simulink model "vibrationAbsorber"  (R2020b)
settings: Solver=VariableStepAuto  StartTime=0.0  StopTime=50  RelTol=1e-3
PreLoadFcn:
  | M1 = 100;
  | K1 = 50;
  | b = 50;
  | K12 = 500;
  | M2 = 5;
settings Model: Creator=Admin  LastModifiedBy=Admin

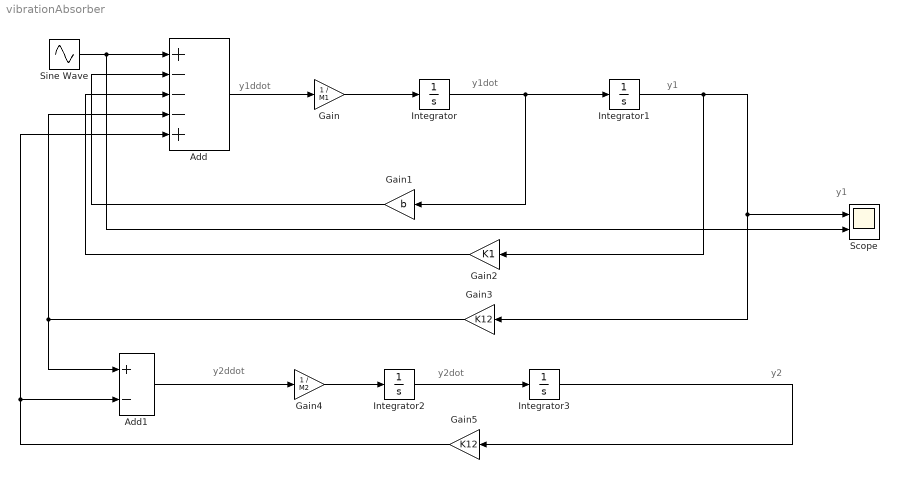
== system vibrationAbsorber ==
  note: y2ddot
  note: y2dot
  note: y1
  note: y1dot
  note: y1ddot
  note: y2
  note: y1
  Add : Sum  Inputs=+---+
  Add1 : Sum  Inputs=+-
  Gain : Gain  Gain=1 / M1
  Gain1 : Gain  Gain=b
  Gain2 : Gain  Gain=K1
  Gain3 : Gain  Gain=K12
  Gain4 : Gain  Gain=1 / M2
  Gain5 : Gain  Gain=K12
  Integrator{,1..3} (4 alike) : Integrator
  Scope : Scope  NumInputPorts=2
  Sine Wave : Sin  Frequency=10  SampleTime=0
  wires:
  Gain5/1 -> Add/5, Add1/2
  Integrator3/1 -> Gain5/1
  Integrator2/1 -> Integrator3/1
  Add1/1 -> Gain4/1
  Gain4/1 -> Integrator2/1
  Integrator/1 -> Gain1/1, Integrator1/1
  Gain1/1 -> Add/2
  Integrator1/1 -> Gain2/1, Scope/1, Gain3/1
  Sine Wave/1 -> Scope/2, Add/1
  Gain/1 -> Integrator/1
  Gain2/1 -> Add/3
  Gain3/1 -> Add/4, Add1/1
  Add/1 -> Gain/1
